simulink model "transmitDBPSK_USRP"  (R2017a)
settings: Solver=VariableStepAuto  StartTime=0.0  StopTime=inf  RelTol=1e-3  EnableMultiTasking=on
values from neighbouring files (symbols this model uses):
  numSymsTot = length(message)    [generateMessage.m]
libraries: commfilt2 x2, commdigbbndpm3 x1, commsdrhw_v2 x1, dspsrcs4 x1
settings Model: Creator=prust  LastModifiedBy=prust
settings OptimizationCC: LifeSpan=inf
settings DebuggingCC: SFUnexpectedBacktrackingDiag=warning  SFNoUnconditionalDefaultTransitionDiag=warning  SFExecutionAtInitializationDiag=none
settings GRTTargetCC: TargetLangStandard=C89/C90 (ANSI)  GeneratePreprocessorConditionals=Disable all
settings ConfigComp: CovMetricSettings=dw  CovHtmlReporting=on  CovSaveCumulativeToWorkspaceVar=on  CovSaveSingleToWorkspaceVar=on  CovExternalEMLEnable=off

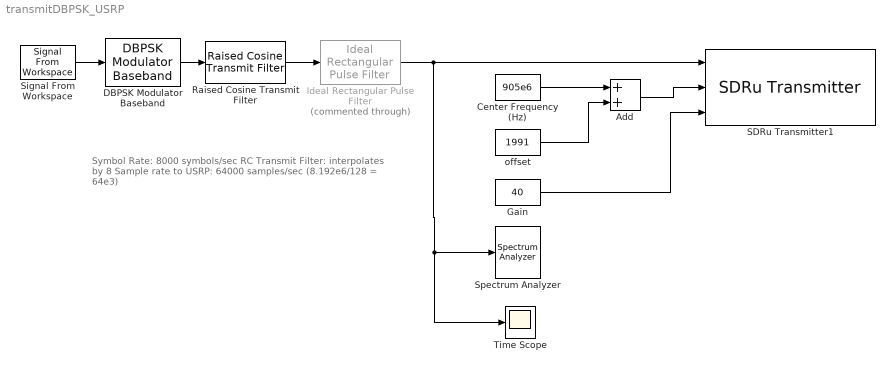
== system transmitDBPSK_USRP ==
  note: Symbol Rate: 8000 symbols/sec
      | RC Transmit Filter: interpolates by 8
      |
      | Sample rate to USRP: 64000 samples/sec
      | (8.192e6/128 = 64e3)
  Add : Sum
  Center Frequency (Hz) : Constant  Value=905e6
  DBPSK Modulator Baseband : commdigbbndpm3/DBPSK Modulator Baseband  Ph=0  outDtype=double
      settings: SourceProductName=Communications System Toolbox  SourceProductBaseCode=CM
  Gain : Constant  Value=40
  Ideal Rectangular Pulse Filter : commfilt2/Ideal Rectangular Pulse Filter  Commented=through  pulseLen=8  pulseDelay=0  InputProcessing=Columns as channels (frame based)  RateOptions=Enforce single-rate processing  sampMode=Mute  normCheck=off  normMode=Sum of samples  filterGain=0.8  saveAsFlag=0  roundingMode=Floor  overflowMode=off  firstCoeffDataTypeStr=Inherit: Same word length as input  firstCoeffMin=[]  firstCoeffMax=[]  firstCoeffLastDataTypeStr=Inherit: Same word length as input  outputDataTypeStr=Inherit: Same as accumulator  outputMin=[]  outputMax=[]  outputLastDataTypeStr=Inherit: Same as accumulator
      settings: SourceProductName=Communications System Toolbox  SourceProductBaseCode=CM
  Raised Cosine Transmit Filter : commfilt2/Raised Cosine Transmit Filter  filtType=Square root  R=.5  filtSpan=4  N=8  filterGain=1  InputProcessing=Columns as channels (frame based)  RateOptions=Enforce single-rate processing  framing=Mute  checkCoeff=off  variableName=rcTxFilt  checkGain=Normalized  sampMode=Mute  saveAsFlag=0  currentFiltSpan=4  D=(4)/2  launchFVT=on  roundingMode=Floor  overflowMode=off  coeffDataTypeStr=Inherit: Same word length as input  coeffMin=[]  coeffMax=[]  coeffLastDataTypeStr=Inherit: Same word length as input  outputDataTypeStr=Inherit: Same as accumulator  outputMin=[]  outputMax=[]  outputLastDataTypeStr=Inherit: Same as accumulator
  SDRu Transmitter1 : commsdrhw_v2/SDRu Transmitter  SourceLibraryInfo="This block requires <a href=\"http://www.mathworks.com/hardware-support/usrp.html\">Communications System Toolbox Support Package for USRP Radio</a>"  rxtx=tx  platform=B200  USRP2_IP='192.168.10.2'  USRP_IP_X300='192.168.10.2'  USRP_IP_X310='192.168.10.2'  USRP_serialNumB200='30703A1'  USRP_serialNumB210=''  ChannelMapping=1  centerFrequency=904e6  centerFrequencySrc=Input port  loOffset=0  loOffsetSrc=Dialog  PPSSource=Internal  clockSource=Internal  masterClkRateB200=8.192e6  masterClkRateB210=32e6  masterClkRateX300=200e6  masterClkRateX310=200e6  masterClkRateParam=8192000  gain=60  gainSrc=Input port  decimInterp=128  decimInterpSrc=Dialog  TransportDataType=int16  USRP2_IP_NUM=[51 48 55 48 51 65 49]  frameLength=362  outputDatatype=Same as transport data type  overrunUnderrunPort=off  sampleTime=1  dboardInfo=|  HOST_DATA_PORT=30000  HOST_CONTROL_PORT=30001  USRP2_DATA_PORT=32769  USRP2_CONTROL_PORT=32768  bufferMode=Continuous streaming  EnableBurstMode=off  NumFramesInBurst=10  USRP_ID='30703A1'
      | dbid: 0
      |           dbName: 'no db found'
      |          freqMin: 0
      |          freqMax: 0
      |          gainMin: 0
      |          gainMax: 0
      |     gainStepSize: 0
      settings: SourceProductName=Communications System Toolbox Support Package for USRP(R) Radio  SourceProductBaseCode=USRP
  Signal From Workspace : dspsrcs4/Signal From Workspace  X=message  Ts=1/8e3  nsamps=numSymsTot*10  OutputAfterFinalValue=Cyclic repetition  ignoreOrWarnInputAndFrameLengths=off  OutputFrames=off
  Spectrum Analyzer : SpectrumAnalyzer
  Time Scope : Scope
  "offset " : Constant  Value=1991
  wires:
  DBPSK Modulator Baseband/1 -> Raised Cosine Transmit Filter/1
  Signal From Workspace/1 -> DBPSK Modulator Baseband/1
  Raised Cosine Transmit Filter/1 -> Ideal Rectangular Pulse Filter/1
  Gain/1 -> SDRu Transmitter1/3
  Center Frequency (Hz)/1 -> Add/1
  "offset "/1 -> Add/2
  Add/1 -> SDRu Transmitter1/2
  Ideal Rectangular Pulse Filter/1 -> Time Scope/1, Spectrum Analyzer/1, SDRu Transmitter1/1
